simulink library "BrickPiSimSubLib_getsensor"  (R2019a)
settings: Solver=VariableStepAuto  StartTime=0.0  StopTime=10.0  RelTol=1e-3
undefined symbols (not defined in the file or in its folder): A
libraries: BrickPiSimSubLib_Read x10, simulink x7, raspberrypilib x4, hdlsllib x3
settings Model: Creator=hahn  LastModifiedBy=uk008555

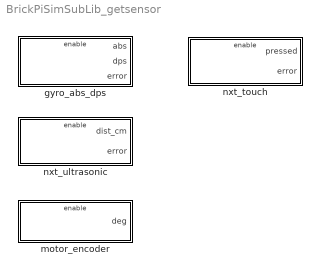
== system BrickPiSimSubLib_getsensor ==
  gyro_abs_dps : Subsystem  mask{Port_Val=1}
      mask prompts: Port_Val "Port"
      mask TypeOptions Port_Val: Port_S/Port_Val
      mask Display: disp(['Get \n EV3_GYRO_ABS_DPS \n Port: ' num2str(Port_Val)])
  motor_encoder : Subsystem  mask{Add_Val=1, Port_Val=A}
      mask prompts: Add_Val "SPI Address"; Port_Val "Port"
      mask init:
      | port_val=Port_Val;
      | switch Port_Val
      |     case 1
      |         port_val='A';
      |     case 2
      |         port_val='B';
      |     case 3
      |         port_val='C';
      |     case 4
      |         port_val='D';
      |     otherwise
      |         port_val='failure';
      | end
      mask TypeOptions Add_Val: Address/Add_Val
      mask TypeOptions Port_Val: Port_M/Port_Val
      mask Display: disp(['Get\n Encoder \n Motor: ' port_val])
  nxt_touch : Subsystem  mask{Port_Val=1}
      mask prompts: Port_Val "Port"
      mask TypeOptions Port_Val: Port_S/Port_Val
      mask Display: disp(['Get \n TOUCH_NXT \n Port: ' num2str(Port_Val)])
  nxt_ultrasonic : Subsystem  mask{Port_Val=1}
      mask prompts: Port_Val "Port"
      mask TypeOptions Port_Val: Port_S/Port_Val
      mask Display: disp(['Get\n NXT_ULTRASONIC \n Port: ' num2str(Port_Val)])

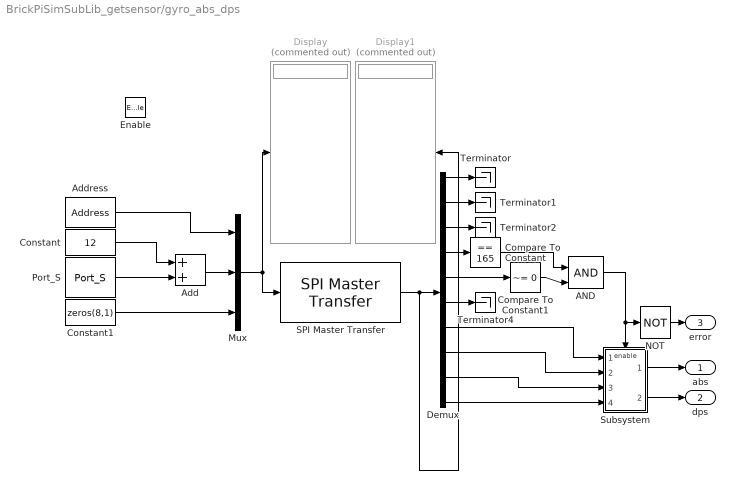
== system BrickPiSimSubLib_getsensor/gyro_abs_dps ==
  Enable : EnablePort
  AND : Logic  IconShape=distinctive  AllPortsSameDT=off  OutDataTypeStr=boolean
  Add : Sum
  Address : BrickPiSimSubLib_Read/Address  Add_Val=1
      settings: SourceProductName=Simulink Support Package for BrickPi
  Compare To Constant : simulink/Logic and Bit Operations/Compare To Constant  relop===  const=165  OutDataTypeStr=boolean
  Compare To Constant1 : simulink/Logic and Bit Operations/Compare To Constant  relop=~=  const=0  OutDataTypeStr=boolean
  Constant : Constant  Value=12  OutDataTypeStr=uint8
  Constant1 : Constant  Value=zeros(8,1)  OutDataTypeStr=uint8
  Demux : Demux  Outputs=10
  Display : Display  Commented=on
  Display1 : Display  Commented=on
  Mux : Mux  Inputs=3
  NOT : Logic  Operator=NOT  IconShape=distinctive  AllPortsSameDT=off  OutDataTypeStr=boolean
  Port_S : BrickPiSimSubLib_Read/Port_S  Port_Val=1
      settings: SourceProductName=Simulink Support Package for BrickPi
  SPI Master Transfer : raspberrypilib/SPI Master Transfer  BoardProperty=Pi 3 Model B+  SPIModule=uint32(0)  Mode=Master  BusSpeed=1000000  Pin=SPI0_CE1  FirstBitToTransfer=Most significant bit (MSB)  ClockMode=0  BlockFunction=Transfer  RegisterAddress=0  OutputDataType=int8  OutputDataLength=1
      settings: SourceProductName=Simulink Support Package for Raspberry Pi Hardware  SourceProductBaseCode=RASPPI
  Subsystem : Subsystem
  Terminator{,1..2,4} (4 alike) : Terminator
  abs : Outport
  dps : Outport  Port=2
  error : Outport  Port=3
  wires:
  Mux/1 -> Display/1, SPI Master Transfer/1
  Port_S/1 -> Add/2
  Constant/1 -> Add/1
  Address/1 -> Mux/1
  Add/1 -> Mux/2
  SPI Master Transfer/1 -> Display1/1, Demux/1
  Demux/1 -> Terminator/1
  Demux/2 -> Terminator1/1
  Demux/3 -> Terminator2/1
  Demux/4 -> Compare To Constant/1
  Compare To Constant/1 -> AND/1
  Demux/6 -> Terminator4/1
  Demux/5 -> Compare To Constant1/1
  Compare To Constant1/1 -> AND/2
  NOT/1 -> error/1
  AND/1 -> NOT/1, Subsystem/Enable
  Demux/7 -> Subsystem/1(In1)
  Demux/8 -> Subsystem/2(In2)
  Demux/9 -> Subsystem/3(In3)
  Demux/10 -> Subsystem/4(In4)
  Subsystem/2(dps) -> dps/1
  Subsystem/1(deg) -> abs/1
  Constant1/1 -> Mux/3

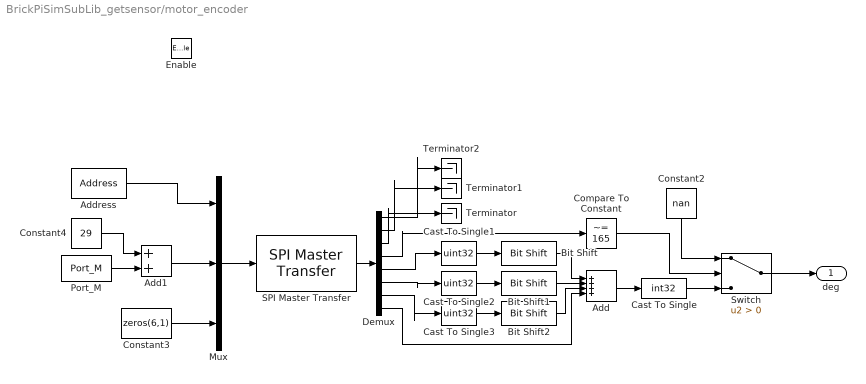
== system BrickPiSimSubLib_getsensor/motor_encoder ==
  Enable : EnablePort
  Add : Sum  Inputs=++++
  Add1 : Sum
  Address : BrickPiSimSubLib_Read/Address  Add_Val=Add_Val
      settings: SourceProductName=Simulink Support Package for BrickPi
  Bit Shift : hdlsllib/Logic and Bit Operations/Bit Shift  mode=Shift Left Logical  N=24
      settings: SourceProductName=Simulink
  Bit Shift1 : hdlsllib/Logic and Bit Operations/Bit Shift  mode=Shift Left Logical  N=16
      settings: SourceProductName=Simulink
  Bit Shift2 : hdlsllib/Logic and Bit Operations/Bit Shift  mode=Shift Left Logical  N=8
      settings: SourceProductName=Simulink
  Cast To Single : DataTypeConversion  OutDataTypeStr=int32
  Cast To Single1 : DataTypeConversion  OutDataTypeStr=uint32
  Cast To Single2 : DataTypeConversion  OutDataTypeStr=uint32
  Cast To Single3 : DataTypeConversion  OutDataTypeStr=uint32
  Compare To Constant : simulink/Logic and Bit Operations/Compare To Constant  relop=~=  const=165  OutDataTypeStr=boolean
  Constant2 : Constant  Value=nan
  Constant3 : Constant  Value=zeros(6,1)  OutDataTypeStr=uint8
  Constant4 : Constant  Value=29  OutDataTypeStr=uint8
  Demux : Demux  Outputs=8
  Mux : Mux  Inputs=3
  Port_M : BrickPiSimSubLib_Read/Port_M  Port_Val=A
      settings: SourceProductName=Simulink Support Package for BrickPi
  SPI Master Transfer : raspberrypilib/SPI Master Transfer  BoardProperty=Pi 3 Model B+  SPIModule=uint32(0)  Mode=Master  BusSpeed=1000000  Pin=SPI0_CE1  FirstBitToTransfer=Most significant bit (MSB)  ClockMode=0  BlockFunction=Transfer  RegisterAddress=0  OutputDataType=int8  OutputDataLength=1
      settings: SourceProductName=Simulink Support Package for Raspberry Pi Hardware  SourceProductBaseCode=RASPPI
  Switch : Switch  Criteria=u2 > Threshold
  Terminator : Terminator
  Terminator1 : Terminator
  Terminator2 : Terminator
  deg : Outport
  wires:
  SPI Master Transfer/1 -> Demux/1
  Demux/7 -> Cast To Single3/1
  Cast To Single/1 -> Switch/3
  Demux/4 -> Compare To Constant/1
  Compare To Constant/1 -> Switch/2
  Constant2/1 -> Switch/1
  Switch/1 -> deg/1
  Constant3/1 -> Mux/3
  Mux/1 -> SPI Master Transfer/1
  Address/1 -> Mux/1
  Port_M/1 -> Add1/2
  Constant4/1 -> Add1/1
  Add1/1 -> Mux/2
  Add/1 -> Cast To Single/1
  Bit Shift1/1 -> Add/2
  Demux/8 -> Add/4
  Bit Shift2/1 -> Add/3
  Bit Shift/1 -> Add/1
  Demux/6 -> Cast To Single2/1
  Demux/5 -> Cast To Single1/1
  Demux/3 -> Terminator/1
  Demux/2 -> Terminator1/1
  Demux/1 -> Terminator2/1
  Cast To Single1/1 -> Bit Shift/1
  Cast To Single2/1 -> Bit Shift1/1
  Cast To Single3/1 -> Bit Shift2/1

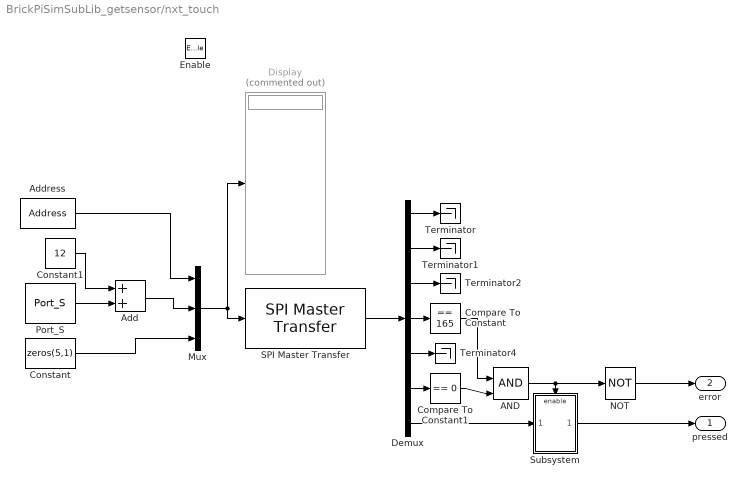
== system BrickPiSimSubLib_getsensor/nxt_touch ==
  Enable : EnablePort
  AND : Logic  IconShape=distinctive  AllPortsSameDT=off  OutDataTypeStr=boolean
  Add : Sum
  Address : BrickPiSimSubLib_Read/Address  Add_Val=1
      settings: SourceProductName=Simulink Support Package for BrickPi
  Compare To Constant : simulink/Logic and Bit Operations/Compare To Constant  relop===  const=165  OutDataTypeStr=boolean
  Compare To Constant1 : simulink/Logic and Bit Operations/Compare To Constant  relop===  const=0  OutDataTypeStr=boolean
  Constant : Constant  Value=zeros(5,1)  OutDataTypeStr=uint8
  Constant1 : Constant  Value=12  OutDataTypeStr=uint8
  Demux : Demux  Outputs=7
  Display : Display  Commented=on
  Mux : Mux  Inputs=3
  NOT : Logic  Operator=NOT  IconShape=distinctive  AllPortsSameDT=off  OutDataTypeStr=boolean
  Port_S : BrickPiSimSubLib_Read/Port_S  Port_Val=1
      settings: SourceProductName=Simulink Support Package for BrickPi
  SPI Master Transfer : raspberrypilib/SPI Master Transfer  BoardProperty=Pi 2 Model B  SPIModule=uint32(0)  Mode=Master  BusSpeed=1000000  Pin=SPI0_CE1  FirstBitToTransfer=Most significant bit (MSB)  ClockMode=0  BlockFunction=Transfer  RegisterAddress=0  OutputDataType=int8  OutputDataLength=1
      settings: SourceProductName=Simulink Support Package for Raspberry Pi Hardware  SourceProductBaseCode=RASPPI
  Subsystem : Subsystem
  Terminator{,1..2,4} (4 alike) : Terminator
  pressed : Outport
  error : Outport  Port=2
  wires:
  Demux/6 -> Compare To Constant1/1
  Demux/4 -> Compare To Constant/1
  Demux/3 -> Terminator2/1
  Add/1 -> Mux/2
  Demux/2 -> Terminator1/1
  Constant/1 -> Mux/3
  Compare To Constant1/1 -> AND/2
  Constant1/1 -> Add/1
  Mux/1 -> Display/1, SPI Master Transfer/1
  Demux/5 -> Terminator4/1
  Demux/1 -> Terminator/1
  SPI Master Transfer/1 -> Demux/1
  Port_S/1 -> Add/2
  AND/1 -> NOT/1, Subsystem/Enable
  Compare To Constant/1 -> AND/1
  NOT/1 -> error/1
  Address/1 -> Mux/1
  Demux/7 -> Subsystem/1(In1)
  Subsystem/1(Out1) -> pressed/1

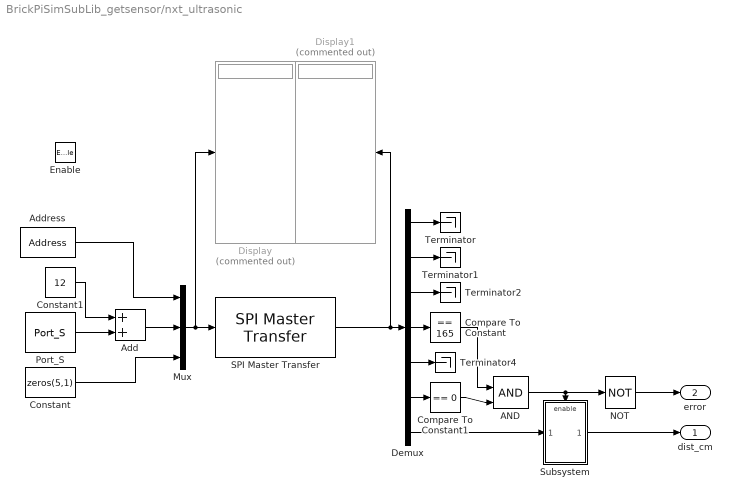
== system BrickPiSimSubLib_getsensor/nxt_ultrasonic ==
  Enable : EnablePort
  AND : Logic  IconShape=distinctive  AllPortsSameDT=off  OutDataTypeStr=boolean
  Add : Sum
  Address : BrickPiSimSubLib_Read/Address  Add_Val=1
      settings: SourceProductName=Simulink Support Package for BrickPi
  Compare To Constant : simulink/Logic and Bit Operations/Compare To Constant  relop===  const=165  OutDataTypeStr=boolean
  Compare To Constant1 : simulink/Logic and Bit Operations/Compare To Constant  relop===  const=0  OutDataTypeStr=boolean
  Constant : Constant  Value=zeros(5,1)  OutDataTypeStr=uint8
  Constant1 : Constant  Value=12  OutDataTypeStr=uint8
  Demux : Demux  Outputs=7
  Display : Display  Commented=on
  Display1 : Display  Commented=on
  Mux : Mux  Inputs=3
  NOT : Logic  Operator=NOT  IconShape=distinctive  AllPortsSameDT=off  OutDataTypeStr=boolean
  Port_S : BrickPiSimSubLib_Read/Port_S  Port_Val=1
      settings: SourceProductName=Simulink Support Package for BrickPi
  SPI Master Transfer : raspberrypilib/SPI Master Transfer  BoardProperty=Pi 2 Model B  SPIModule=uint32(0)  Mode=Master  BusSpeed=1000000  Pin=SPI0_CE1  FirstBitToTransfer=Most significant bit (MSB)  ClockMode=0  BlockFunction=Transfer  RegisterAddress=0  OutputDataType=int8  OutputDataLength=1
      settings: SourceProductName=Simulink Support Package for Raspberry Pi Hardware  SourceProductBaseCode=RASPPI
  Subsystem : Subsystem
  Terminator{,1..2,4} (4 alike) : Terminator
  dist_cm : Outport
  error : Outport  Port=2
  wires:
  NOT/1 -> error/1
  AND/1 -> Subsystem/Enable, NOT/1
  Constant/1 -> Mux/3
  Subsystem/1(value) -> dist_cm/1
  Demux/7 -> Subsystem/1(In1)
  Compare To Constant/1 -> AND/1
  Demux/6 -> Compare To Constant1/1
  Constant1/1 -> Add/1
  Demux/1 -> Terminator/1
  Mux/1 -> SPI Master Transfer/1, Display/1
  Demux/5 -> Terminator4/1
  Address/1 -> Mux/1
  Port_S/1 -> Add/2
  Compare To Constant1/1 -> AND/2
  Add/1 -> Mux/2
  Demux/2 -> Terminator1/1
  SPI Master Transfer/1 -> Display1/1, Demux/1
  Demux/4 -> Compare To Constant/1
  Demux/3 -> Terminator2/1

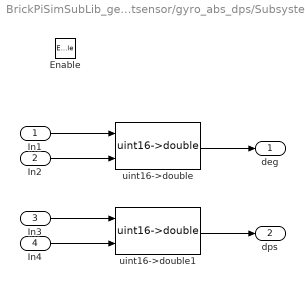
== system BrickPiSimSubLib_getsensor/gyro_abs_dps/Subsystem ==
  In1 : Inport
  In2 : Inport  Port=2
  In3 : Inport  Port=3
  In4 : Inport  Port=4
  Enable : EnablePort
  uint16->double : BrickPiSimSubLib_Read/uint16->double  SystemSampleTime=-1
      settings: SourceProductName=Simulink Support Package for BrickPi
  uint16->double1 : BrickPiSimSubLib_Read/uint16->double  SystemSampleTime=-1
      settings: SourceProductName=Simulink Support Package for BrickPi
  deg : Outport
  dps : Outport  Port=2
  wires:
  In1/1 -> uint16->double/1
  In2/1 -> uint16->double/2
  uint16->double/1 -> deg/1
  In3/1 -> uint16->double1/1
  In4/1 -> uint16->double1/2
  uint16->double1/1 -> dps/1

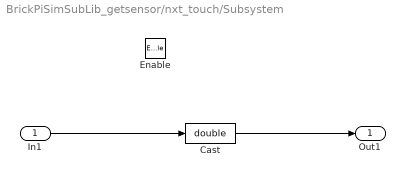
== system BrickPiSimSubLib_getsensor/nxt_touch/Subsystem ==
  In1 : Inport
  Enable : EnablePort
  Cast : DataTypeConversion  OutDataTypeStr=double
  Out1 : Outport
  wires:
  In1/1 -> Cast/1
  Cast/1 -> Out1/1

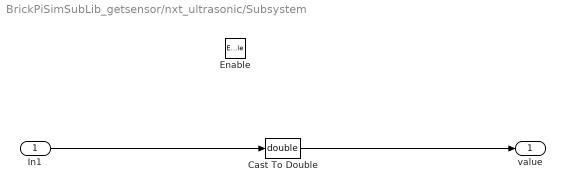
== system BrickPiSimSubLib_getsensor/nxt_ultrasonic/Subsystem ==
  In1 : Inport
  Enable : EnablePort
  Cast To Double : DataTypeConversion  OutDataTypeStr=double
  value : Outport
  wires:
  In1/1 -> Cast To Double/1
  Cast To Double/1 -> value/1
